simulink model "ApenasDelay"  (Simulink 8.2)
settings: Solver=ode4  SolverMode=SingleTasking  StartTime=0.0  StopTime=300  FixedStep=0.01  RelTol=1e-3
InitFcn:
  | Main;
undefined symbols (not defined in the file or in its folder): A, B, C, Csimulink, Dsimulink, T, zk0
settings Model: Creator=Kawakami  LastModifiedBy=Eduardo
settings DataIOCC: LimitDataPoints=off  SaveOutput=off  SaveTime=off  TimeSaveName=t  SignalLoggingName=sigsOut
settings OptimizationCC: BooleanDataType=off
settings DebuggingCC: SaveWithParameterizedLinksMsg=none  SignalResolutionControl=TryResolveAllWithWarning  SolverPrmCheckMsg=none  MultiTaskDSMMsg=warning  MultiTaskCondExecSysMsg=none
settings HardwareCC: TargetUnknown=on
settings RTWCC: IncludeERTFirstTime=on

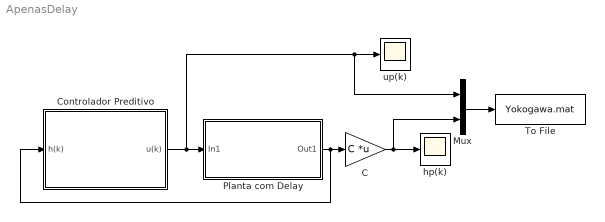
== system ApenasDelay ==
  C : Gain  Gain=C  Multiplication=Matrix(K*u)  SampleTime=T
  "Controlador Preditivo  " : Subsystem
  Mux : Mux  Inputs=2
  "Planta com Delay " : Subsystem
  To File : ToFile  Filename=Yokogawa.mat  MatrixName=Yokogawa  SampleTime=T
  hp(k) : Scope
      settings: YMin=-1.25  YMax=2.25
  up(k) : Scope
      settings: TimeRange=100  YMin=-4  YMax=1.25
  wires:
  Mux/1 -> To File/1
  "Controlador Preditivo  "/1(u(k)) -> Mux/1, up(k)/1, "Planta com Delay "/1(In1)
  "Planta com Delay "/1(Out1) -> "Controlador Preditivo  "/1(h(k)), C/1
  C/1 -> Mux/2, hp(k)/1

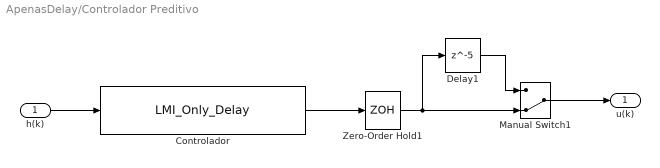
== system ApenasDelay/Controlador Preditivo   ==
  h(k) : Inport
  Controlador : S-Function  FunctionName=LMI_Only_Delay  Parameters=Adelay, Bdelay, Cdelay, tao, Smeio, Rmeio, Umax, T  EnableBusSupport=off
  Delay1 : Delay  DelayLength=5  SampleTime=T
  Manual Switch1 : ManualSwitch  CurrentSetting=0
  Zero-Order Hold1 : ZeroOrderHold  SampleTime=T
  u(k) : Outport
  wires:
  h(k)/1 -> Controlador/1
  Delay1/1 -> Manual Switch1/1
  Zero-Order Hold1/1 -> Manual Switch1/2, Delay1/1
  Manual Switch1/1 -> u(k)/1
  Controlador/1 -> Zero-Order Hold1/1

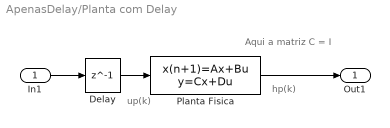
== system ApenasDelay/Planta com Delay  ==
  note: Aqui a matriz C = I
  note: up(k)
  note: hp(k)
  In1 : Inport
  Delay : Delay  DelayLength=1  SampleTime=T
  "Planta Fisica " : DiscreteStateSpace  A=A  B=B  C=Csimulink  D=Dsimulink  X0=zk0  SampleTime=T
  Out1 : Outport
  wires:
  Delay/1 -> "Planta Fisica "/1
  In1/1 -> Delay/1
  "Planta Fisica "/1 -> Out1/1
